simulink model "MSD_modelrefrence"  (R2016a)
settings: Solver=VariableStepAuto  StartTime=0.0  StopTime=30  RelTol=1e-3
libraries: neural x2
settings Model: Creator=Hamid  LastModifiedBy=Hamid

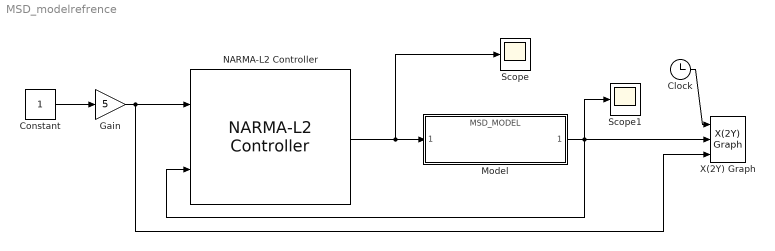
== system MSD_modelrefrence ==
  Clock : Clock
  Constant : Constant
  Gain : Gain  Gain=5
  Model : ModelReference  ModelNameDialog=MSD_MODEL.slx  SimulationMode=Normal  ModelReferenceVersion=1.1
  NARMA-L2 Controller : neural/Control Systems/NARMA-L2 Controller  Normalize=1  IW1_1=[-3.0864508724970836;-1.9719335170338737;1.6361019297287174;1.50266039128699;-4.2149867624528268;-3.4627382333477046]  IW3_2=[-8.5681034588004561;7.7634427146936016;6.4631959948233364;-9.6798176543915773;8.3808893815291725;8.3886711923852868]  IW5_3=-0.8166084733131701  LW2_1=[1.0608345505122336 1.5887617567946724 -2.126810169233015 -3.4424164679617988 0.16228980868785187 1.0041215300280237]  LW4_3=[-3.1433741420621408 2.8276758198347509 2.0075302171971035 7.979059261841992 -5.0188947326120763 -2.7373150562188795]  LW5_4=0.37668860774795709  LW6_5=0.00030183263797240416  LW6_2=-0.14800374527064342  B1=[3.318678405247967;1.428848310972104;-0.37904562270201342;0.7684672522432473;-3.2613490356932813;-3.8366903052847601]  B2=0.14361854365818646  B3=[8.2250306560299666;-6.3526769115335995;-5.9549186484922787;-2.7946229708318735;5.9169106983543598;8.4120618736570716]  B4=-2.7799860669729535  Limit_output=0  min_output=-Inf  max_output=Inf  Use_Previous_Weights=1  Ts=0.01  S1=6  Ni=1  Nj=1  sim_file=MSD_MODEL  trainfun=trainlm  Use_validation=1  Use_Testing=1  max_i=150  min_i=-150  max_i_int=30  min_i_int=0.1  sam_training=15000  epochs=1000  minp=-147.74777877201481  maxp=133.80611261842739  mint=-13.454369454109161  maxt=133.80611261842739
  Scope : Scope
  Scope1 : Scope
  X(2Y) Graph : neural/Control Systems/X(2Y)  Graph  xmin=0  xmax=5  ymin=21  ymax=22  st=-1
  wires:
  NARMA-L2 Controller/1 -> Model/1, Scope/1
  Model/1 -> NARMA-L2 Controller/2, X(2Y) Graph/2, Scope1/1
  Constant/1 -> Gain/1
  Gain/1 -> NARMA-L2 Controller/1, X(2Y) Graph/3
  Clock/1 -> X(2Y) Graph/1
